simulink model "force_simulation_model"  (R2023a)
settings: Solver=VariableStepAuto  StartTime=0.0  StopTime=10.0  RelTol=1e-3
libraries: simulink x1
settings Model: Creator=s202421  LastModifiedBy=s202421

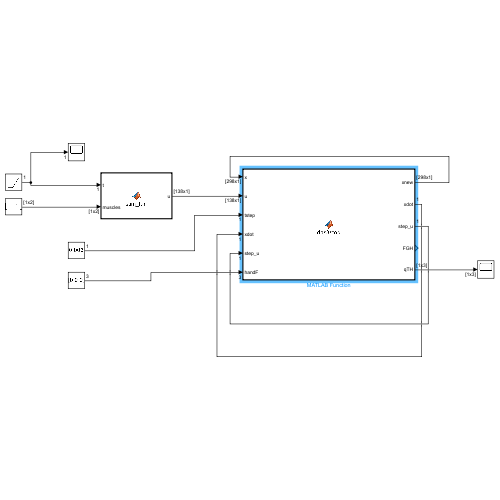
[thumbnail: Simulink's stored preview of the top-level diagram]
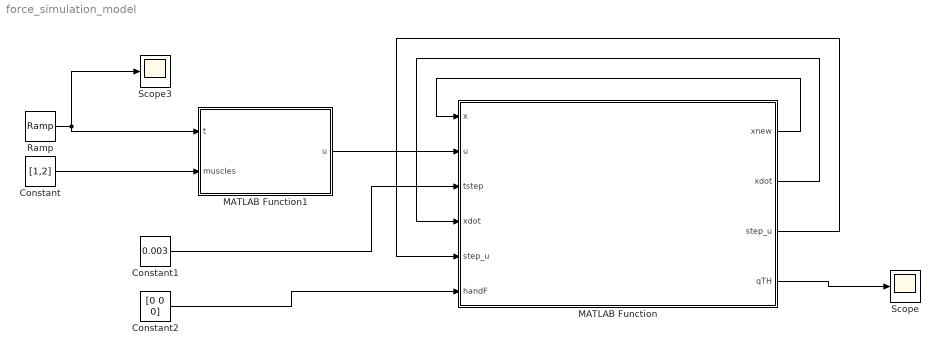
== system force_simulation_model ==
  Constant : Constant  Value=[1,2]  VectorParams1D=off
  Constant1 : Constant  Value=0.003
  Constant2 : Constant  Value=[0 0 0]
  MATLAB Function : MATLAB Function  TreatAsAtomicUnit=on
  MATLAB Function1 : MATLAB Function  TreatAsAtomicUnit=on
  Ramp : simulink/Sources/Ramp  slope=1  start=0  InitialOutput=0
  Scope : Scope
  Scope3 : Scope
  wires:
  MATLAB Function/1(xnew) -> MATLAB Function/1(x)
  Ramp/1 -> MATLAB Function1/1(t), Scope3/1
  Constant/1 -> MATLAB Function1/2(muscles)
  MATLAB Function1/1(u) -> MATLAB Function/2(u)
  MATLAB Function/3(step_u) -> MATLAB Function/5("step_u ")
  MATLAB Function/2(xdot) -> MATLAB Function/4("xdot ")
  Constant1/1 -> MATLAB Function/3(tstep)
  Constant2/1 -> MATLAB Function/6(handF)
  MATLAB Function/4(qTH) -> Scope/1

== matlab function force_simulation_model/MATLAB Function1 ==
  data: t input; u output; muscles input
function u  = stim_fun(t, muscles)
    nmus = 138;
    u = zeros(nmus,1);
    %u = 0;
    if muscles ~= 0
        if t > 2.5
            u(muscles) = 1;
            %u = 1;
        end 
        if t > 5
            u(muscles)=0;
            %u = 0;
        end
    end
end

== matlab function force_simulation_model/MATLAB Function ==
  data: x input double size=[298 1]; u input double size=[138 1]; xnew output double size=[298 1]; tstep input; xdot input double size=[298 1]; step_u input double size=[138 1]; xdot output; step_u output; qTH output double size=[3 1]; handF input double size=[3 1]
function [xnew, xdot, step_u, qTH] = das3step(x, u, tstep, xdot, step_u, handF)
    coder.extrinsic('das3')
    M = zeros(5,1);
    exF = zeros(2,1);
    
    f = zeros(298,1);
    qTH = zeros(3,1);
    dfdu = zeros(298,138);
    dfdu = sparse(dfdu);

    dfdx = zeros(298,298);
    dfdx = sparse(dfdx);

    dfdxdot = dfdx;
    [f, dfdx, dfdxdot, dfdu, ~,~,qTH] = das3('Dynamics',xdot,step_u,M,exF,handF);
    dfdx = sparse(dfdx);
    dfdx = full(dfdx);
    dfdxdot = full(dfdxdot);
    dfdu = full(dfdu);
	% Solve the change in x from the 1st order Rosenbrock formula
	du = u - step_u;
	dx = (dfdx + dfdxdot/tstep)\(dfdxdot*xdot - f - dfdu*du);
	xnew = x + dx;
	
	% update variables for the next simulation step
	xdot = dx/tstep;
	step_u = u;

end
